simulink model "Citation"  (R2018a)
settings: Solver=ode5  StartTime=0.0  StopTime=500  FixedStep=0.01  RelTol=1e-3  EnableMultiTasking=on
InitFcn:
  | initcit
values from neighbouring files (symbols this model uses):
  aeroinit = [dp_ini;inicoef('CX0');inicoef('CXa');inicoef('CXa2');inicoef('CXq')     ;inicoef('CXde');inicoef('CY0');inicoef('CYB');inicoef('CYp');inicoef('CYr')     ;inicoef('CYda');inicoef('CYdr');inicoef('CZ0');inicoef('CZa');inicoef('CZq')     ;inicoef('CZde');inicoef('Cl0');inicoef('ClB');inicoef('Clp');inicoef('Clr')     ;inicoef('Clda');inicoef('Cldr');inicoef('Cm0');inicoef('Cma');inicoef('Cmq')     ; ...(+113 chars)    [initcit.m]
  h_l_old = zeros(6,sample_size)    [initcit.m]
  h_m_old = zeros(4,sample_size)    [initcit.m]
  h_n_old = zeros(6,sample_size)    [initcit.m]
  h_X_old = zeros(5,sample_size)    [initcit.m]
  h_Y_old = zeros(6,sample_size)    [initcit.m]
  h_Z_old = zeros(4,sample_size)    [initcit.m]
  I = [massinit(5),0, -massinit(8);0, massinit(6),0;-massinit(8),0, massinit(7)]    [initcit.m]
  p_l = [inicoef('Cl0');inicoef('ClB');inicoef('Clp');inicoef('Clr')     ;inicoef('Clda');inicoef('Cldr')].*ones(6,sample_size)    [initcit.m]
  p_m = [inicoef('Cm0');inicoef('Cma');inicoef('Cmq')     ;inicoef('Cmde')].*ones(4,sample_size)    [initcit.m]
  p_n = 0.71*ones(6,sample_size)    [initcit.m]
  p_X = [inicoef('CX0');inicoef('CXa');inicoef('CXa2');inicoef('CXq')     ;inicoef('CXde')].*ones(5,sample_size)    [initcit.m]
  p_Y = [inicoef('CY0');inicoef('CYB');inicoef('CYp');inicoef('CYr')     ;inicoef('CYda');inicoef('CYdr')].*ones(6,sample_size)    [initcit.m]
  p_Z = [inicoef('CZ0');inicoef('CZa');inicoef('CZq')     ;inicoef('CZde')].*ones(4,sample_size)    [initcit.m]
  Pcov_l = 10000*eye(6)    [initcit.m]
  Pcov_m = 10000*eye(4)    [initcit.m]
  Pcov_n = 10000*eye(6)    [initcit.m]
  Pcov_X = 10000*eye(5)    [initcit.m]
  Pcov_Y = 10000*eye(6)    [initcit.m]
  Pcov_Z = 10000*eye(4)    [initcit.m]
  T0 = 288.15    [rho_test.m]
  Vw915 = 0    [initcit.m]
  winddir = 45*(pi/180)    (= 0.785398163397)    [initcit.m]
  x0 = []    [cessnac550_3d_sfnc.m]    (also in sfunxyauto.m)
  y_l = zeros(1,sample_size)    [initcit.m]
  y_l_est_old = zeros(size(y_l))    [initcit.m]
  y_m = zeros(1,sample_size)    [initcit.m]
  y_m_est_old = zeros(size(y_m))    [initcit.m]
  y_n = zeros(1,sample_size)    [initcit.m]
  y_n_est_old = zeros(size(y_n))    [initcit.m]
  y_X = zeros(1,sample_size)    [initcit.m]
  y_X_est_old = zeros(size(y_X))    [initcit.m]
  y_Y = zeros(1,sample_size)    [initcit.m]
  y_Y_est_old = zeros(size(y_Y))    [initcit.m]
  y_Z = zeros(1,sample_size)    [initcit.m]
  y_Z_est_old = zeros(size(y_Z))    [initcit.m]
undefined symbols (not defined in the file or in its folder): chord, cv1, cv2, cv3, cv4, deltagmax1, deltagmax2, deltagmax3, deltagmax4, Deng, ealphag, ealphas, g0, hDME, hGS, kt1, kt2, kt3, lh, massinit, matbuaf, matdaf, matdam, matdbbf, matdeaf, matdgaf, matdqaf, matduaf, matdwaw, matedhr, mateif, matelhr, matemhr, matemv1, matemv2, matemve, matetam, mateuaf, matfaaf, matfaxl, matff, matibaf, matibb, matibmh, matipaf, matipmh, matiraf, matiuaf, matiwaf, matlaf, matlam, matleaf, matleam, matlgaf, matlqaf, matluaf, matmaaf, matmaam, matmaf, matmam ... (+75)
libraries: simulink x5, templibrary x3, vrlib x1
(part 2 of 6)

== system Citation/Aero Forces & Moments /Aerodynamic Moment Components/Cm ==
  "model output " : Inport
  Dynamic Pressure : Inport  Port=2
  Constant : Constant  Value=massinit
  Constant1 : Constant  Value=S
  Constant2 : Constant  Value=chord
  Demux2 : Demux  Outputs=[1 1 1 9 1 1 1 22]
  Demux3 : Demux  Outputs=[4 1 1 1 1]
  Divide : Product  Inputs=*/
  Product : Product  Inputs=3
  Product{1,3..5} (4 alike) : Product
  Product2 : Product  Inputs=3
  Sum : Sum  Inputs=|+++
  Sum1 : Sum  Inputs=|+-
  Sum2 : Sum  Inputs=|+-
  Terminator{1..6} (6 alike) : Terminator
  Cm : Outport
  wires:
  Demux3/4 -> Sum1/2  "Izz"
  Demux2/8 -> Terminator4/1
  Demux3/5 -> Product5/2  "Ixz"
  Demux2/7 -> Terminator6/1  "rdot"
  Demux2/1 -> Product3/2, Product3/1, Product2/1  "p"
  Demux2/6 -> Product1/1  "qdot"
  Demux3/2 -> Sum1/1  "Ixx"
  Demux2/4 -> Terminator3/1
  Demux3/1 -> Terminator5/1
  Demux2/5 -> Terminator2/1  "pdot"
  Demux3/3 -> Product1/2  "Iyy"
  "model output "/1 -> Demux2/1
  Constant/1 -> Demux3/1
  Sum/1 -> Divide/1
  Divide/1 -> Cm/1
  Dynamic Pressure/1 -> Product/1
  Constant1/1 -> Product/2
  Constant2/1 -> Product/3
  Product/1 -> Divide/2
  Product1/1 -> Sum/2  "qdot*Iyy"
  Sum1/1 -> Product2/3
  Demux2/2 -> Terminator1/1  "q"
  Demux2/3 -> Product4/2, Product4/1, Product2/2  "r"
  Product2/1 -> Sum/1  "rp*(Ixx-Izz)"
  Product3/1 -> Sum2/1  "p^2"
  Product4/1 -> Sum2/2  "r^2"
  Sum2/1 -> Product5/1
  Product5/1 -> Sum/3  "(p^2 - r^2)*(Ixz)"

== system Citation/Aero Forces & Moments /Aerodynamic Moment Components/Cn ==
  model output : Inport
  Dynamic Pressure : Inport  Port=2
  Constant : Constant  Value=massinit
  Constant1 : Constant  Value=S
  Constant2 : Constant  Value=span
  Demux2 : Demux  Outputs=[1 1 1 9 1 1 1 22]
  Demux3 : Demux  Outputs=[4 1 1 1 1]
  Divide : Product  Inputs=*/
  Product : Product  Inputs=3
  Product1 : Product
  Product2 : Product  Inputs=3
  Product3 : Product
  Product4 : Product
  Sum : Sum  Inputs=+++
  Sum1 : Sum  Inputs=|-+
  Sum2 : Sum  Inputs=|+-
  Terminator{1,3..5} (4 alike) : Terminator
  Cn : Outport
  wires:
  Demux3/4 -> Product1/2  "Izz"
  Demux2/8 -> Terminator4/1
  Demux3/5 -> Product3/2  "Ixz"
  Demux2/2 -> Product4/1, Product2/2  "q"
  Demux2/7 -> Product1/1  "rdot"
  Demux2/6 -> Terminator1/1  "qdot"
  Demux3/2 -> Sum1/1  "Ixx"
  Demux2/4 -> Terminator3/1
  Demux3/1 -> Terminator5/1
  Demux2/5 -> Sum2/2  "pdot"
  Demux3/3 -> Sum1/2  "Iyy"
  model output/1 -> Demux2/1
  Constant/1 -> Demux3/1
  Dynamic Pressure/1 -> Product/1
  Constant1/1 -> Product/2
  Constant2/1 -> Product/3
  Product/1 -> Divide/2  "0.5*rho*V^2*S*b"
  Sum/1 -> Divide/1  "rdot*Izz+pq*(Iyy-Ixx)+(qr-pdot)*Ixz"
  Product1/1 -> Sum/2  "rdot*Izz"
  Demux2/1 -> Product2/1  "p"
  Demux2/3 -> Product4/2  "r"
  Sum1/1 -> Product2/3
  Product2/1 -> Sum/1  "p*q*(Iyy-Ixx)"
  Product3/1 -> Sum/3  "Ixz*(qr-pdot)"
  Product4/1 -> Sum2/1
  Sum2/1 -> Product3/1
  Divide/1 -> Cn/1

== system Citation/Aerodynamic Parameter Estimation/Statistics 2/Auto_correlation ==
  delta_window : Inport
  kgap : Inport  Port=2
  Memory3 : Memory
  Memory4 : Memory
  autocorrelation : MATLAB Function  TreatAsAtomicUnit=on
  PI_kgap : Outport
  PI_kgap_avg : Outport  Port=2
  wires:
  kgap/1 -> autocorrelation/2(kgap)
  autocorrelation/3(counter) -> Memory4/1
  Memory4/1 -> autocorrelation/4("counter ")
  autocorrelation/1(PI_kgap) -> PI_kgap/1
  autocorrelation/2(kgap_avg) -> Memory3/1, PI_kgap_avg/1
  Memory3/1 -> autocorrelation/3("kgap_avg ")
  delta_window/1 -> autocorrelation/1(delta)

== system Citation/Aerodynamic Parameter Estimation/Statistics 2/variance ==
  delta : Inport
  MATLAB Function : MATLAB Function  TreatAsAtomicUnit=on
  Memory : Memory
  Memory1 : Memory
  Memory2 : Memory  InitialCondition=[0, 0]
  variance : Outport
  sigma_avg : Outport  Port=2
  wires:
  Memory1/1 -> MATLAB Function/2("delta_avg ")
  MATLAB Function/4(sigma_avg) -> sigma_avg/1, Memory2/1
  Memory2/1 -> MATLAB Function/4("sigma_avg ")
  MATLAB Function/2(delta_avg) -> Memory1/1  "average"
  Memory/1 -> MATLAB Function/3("counter ")
  MATLAB Function/1(var) -> variance/1
  MATLAB Function/3(counter) -> Memory/1
  delta/1 -> MATLAB Function/1(delta)

== system Citation/Aerodynamic Parameter Estimation/Statistics 3/Auto_correlation ==
  delta_window : Inport
  kgap : Inport  Port=2
  Memory3 : Memory
  Memory4 : Memory
  autocorrelation : MATLAB Function  TreatAsAtomicUnit=on
  PI_kgap : Outport
  PI_kgap_avg : Outport  Port=2
  wires:
  delta_window/1 -> autocorrelation/1(delta)
  Memory3/1 -> autocorrelation/3("kgap_avg ")
  autocorrelation/2(kgap_avg) -> PI_kgap_avg/1, Memory3/1
  autocorrelation/1(PI_kgap) -> PI_kgap/1
  Memory4/1 -> autocorrelation/4("counter ")
  autocorrelation/3(counter) -> Memory4/1
  kgap/1 -> autocorrelation/2(kgap)

== system Citation/Aerodynamic Parameter Estimation/Statistics 3/variance ==
  delta : Inport
  MATLAB Function : MATLAB Function  TreatAsAtomicUnit=on
  Memory : Memory
  Memory1 : Memory
  Memory2 : Memory  InitialCondition=[0, 0]
  variance : Outport
  sigma_avg : Outport  Port=2
  wires:
  delta/1 -> MATLAB Function/1(delta)
  MATLAB Function/3(counter) -> Memory/1
  MATLAB Function/1(var) -> variance/1
  Memory/1 -> MATLAB Function/3("counter ")
  MATLAB Function/2(delta_avg) -> Memory1/1  "average"
  Memory2/1 -> MATLAB Function/4("sigma_avg ")
  MATLAB Function/4(sigma_avg) -> Memory2/1, sigma_avg/1
  Memory1/1 -> MATLAB Function/2("delta_avg ")

== system Citation/Aerodynamic Parameter Estimation/Statistics 4/Auto_correlation ==
  delta_window : Inport
  kgap : Inport  Port=2
  Memory3 : Memory
  Memory4 : Memory
  autocorrelation : MATLAB Function  TreatAsAtomicUnit=on
  PI_kgap : Outport
  PI_kgap_avg : Outport  Port=2
  wires:
  kgap/1 -> autocorrelation/2(kgap)
  autocorrelation/3(counter) -> Memory4/1
  Memory4/1 -> autocorrelation/4("counter ")
  autocorrelation/1(PI_kgap) -> PI_kgap/1
  autocorrelation/2(kgap_avg) -> Memory3/1, PI_kgap_avg/1
  Memory3/1 -> autocorrelation/3("kgap_avg ")
  delta_window/1 -> autocorrelation/1(delta)

== system Citation/Aerodynamic Parameter Estimation/Statistics 4/variance ==
  delta : Inport
  MATLAB Function : MATLAB Function  TreatAsAtomicUnit=on
  Memory : Memory
  Memory1 : Memory
  Memory2 : Memory  InitialCondition=[0, 0]
  variance : Outport
  sigma_avg : Outport  Port=2
  wires:
  Memory1/1 -> MATLAB Function/2("delta_avg ")
  MATLAB Function/4(sigma_avg) -> sigma_avg/1, Memory2/1
  Memory2/1 -> MATLAB Function/4("sigma_avg ")
  MATLAB Function/2(delta_avg) -> Memory1/1  "average"
  Memory/1 -> MATLAB Function/3("counter ")
  MATLAB Function/1(var) -> variance/1
  MATLAB Function/3(counter) -> Memory/1
  delta/1 -> MATLAB Function/1(delta)

== system Citation/Cessna Citation 500/Actuators/da ==
  In : Inport
  Gain : Gain  Gain=13  SaturateOnIntegerOverflow=on  OutDataTypeStr=Inherit: Same as input  ParamDataTypeStr=Inherit: Same as input
  Integrator : Integrator  InitialCondition=u0(2)
  Sum : Sum  Inputs=|+-  SaturateOnIntegerOverflow=on
  Out : Outport
  wires:
  Integrator/1 -> Out/1, Sum/2
  In/1 -> Sum/1
  Sum/1 -> Gain/1
  Gain/1 -> Integrator/1

== system Citation/Cessna Citation 500/Actuators/de ==
  In : Inport
  Gain : Gain  Gain=13  SaturateOnIntegerOverflow=on  OutDataTypeStr=Inherit: Same as input  ParamDataTypeStr=Inherit: Same as input
  Integrator : Integrator  InitialCondition=u0(1)
  Sum : Sum  Inputs=|+-  SaturateOnIntegerOverflow=on
  Out : Outport
  wires:
  Integrator/1 -> Out/1, Sum/2
  In/1 -> Sum/1
  Sum/1 -> Gain/1
  Gain/1 -> Integrator/1

== system Citation/Cessna Citation 500/Actuators/dr ==
  In : Inport
  Gain : Gain  Gain=13  SaturateOnIntegerOverflow=on  OutDataTypeStr=Inherit: Same as input  ParamDataTypeStr=Inherit: Same as input
  Integrator : Integrator  InitialCondition=u0(3)
  Sum : Sum  Inputs=|+-  SaturateOnIntegerOverflow=on
  Out : Outport
  wires:
  Integrator/1 -> Out/1, Sum/2
  In/1 -> Sum/1
  Sum/1 -> Gain/1
  Gain/1 -> Integrator/1

== system Citation/Cessna Citation 500/Actuators/flaps ==
  In : Inport
  Gain : Gain  Gain=0.9  SaturateOnIntegerOverflow=on  OutDataTypeStr=Inherit: Same as input  ParamDataTypeStr=Inherit: Same as input
  Integrator : Integrator  InitialCondition=u0(7)
  Sum : Sum  Inputs=|+-  SaturateOnIntegerOverflow=on
  Out : Outport
  wires:
  Integrator/1 -> Out/1, Sum/2
  In/1 -> Sum/1
  Sum/1 -> Gain/1
  Gain/1 -> Integrator/1

== system Citation/Cessna Citation 500/Actuators/gear ==
  In : Inport
  Gain : Gain  Gain=0.6  SaturateOnIntegerOverflow=on  OutDataTypeStr=Inherit: Same as input  ParamDataTypeStr=Inherit: Same as input
  Integrator : Integrator  InitialCondition=u0(8)
  Sum : Sum  Inputs=|+-  SaturateOnIntegerOverflow=on
  Out : Outport
  wires:
  Integrator/1 -> Out/1, Sum/2
  In/1 -> Sum/1
  Sum/1 -> Gain/1
  Gain/1 -> Integrator/1

== system Citation/Cessna Citation 500/Citation model DASMAT/AIRCRAFT MODEL ==
  ua : Inport
  ut : Inport  Port=2
  massinit : Inport  Port=3
  Environment : Inport  Port=4
  AFM : Subsystem
  AIRDATA : Subsystem
  Demux : Demux  Outputs=[8 1]
  EFM : Subsystem
  EQM : Subsystem
  FM SORT : Subsystem
  GRAVITY : Subsystem
  LANDING GEAR : Subsystem
  OBSERVATIONS : Subsystem
  WIND/TURBULENCE : Subsystem
  x : Outport
  xdot : Outport  Port=2
  yatm : Outport  Port=3
  yad1 : Outport  Port=4
  yad2 : Outport  Port=5
  wind : Outport  Port=6
  gust : Outport  Port=7
  yacc : Outport  Port=8
  yfp : Outport  Port=9
  ys : Outport  Port=10
  FMa : Outport  Port=11
  FMag : Outport  Port=12
  FMt : Outport  Port=13
  ypp : Outport  Port=14
  wires:
  AFM/1(FMa) -> FM SORT/1(FMa), EQM/2(FMa)
  OBSERVATIONS/3(ys) -> ys/1
  OBSERVATIONS/2(yfp) -> yfp/1
  EQM/4(FMtot corrected) -> OBSERVATIONS/4(FMtot)
  EQM/3(yuvw) -> OBSERVATIONS/3(yuvw)
  EFM/1(FMt) -> FM SORT/3(FMt), FMt/1
  AFM/4(FMag) -> FM SORT/2(FMag), FMag/1
  ua/1 -> AFM/2(ua), LANDING GEAR/4(ua)
  ut/1 -> EFM/2(ut)
  OBSERVATIONS/1(yacc) -> yacc/1
  FM SORT/1(FMtot) -> EQM/1("FMtot ")
  EQM/5(FMa corrected) -> OBSERVATIONS/5(FMa), FMa/1
  AFM/2(FMadot) -> EQM/3(FMadot)
  AFM/3(FMbdot) -> EQM/4(FMbdot)
  GRAVITY/1(Fgr) -> FM SORT/4("Fgr "), OBSERVATIONS/6(Fgr)
  massinit/1 -> EFM/3(massinit), AFM/3(massinit), GRAVITY/2(massinit), EQM/5(massinit), OBSERVATIONS/7(massinit), LANDING GEAR/3(massinit)
  AIRDATA/3(yad2) -> EFM/6(yad2), AFM/5(yad2), yad2/1
  AIRDATA/2(yad1) -> AFM/4(yad1), EFM/5(yad1), yad1/1
  AIRDATA/1(yatm) -> yatm/1, GRAVITY/3(yatm), OBSERVATIONS/8(yatm), EFM/4(yatm), AFM/7(yatm)
  EQM/1(x) -> GRAVITY/1("x "), LANDING GEAR/1(x), EFM/1(x), AFM/1(x), WIND/TURBULENCE/1("x "), AIRDATA/1(x), x/1, OBSERVATIONS/1(x)
  WIND/TURBULENCE/1(wind) -> EQM/6(wind), wind/1
  EQM/2(xdot) -> xdot/1, OBSERVATIONS/2(xdot), LANDING GEAR/2(xdot)
  Environment/1 -> Demux/1
  Demux/1 -> gust/1, AFM/6(gust)
  Demux/2 -> AIRDATA/2(terrain elevation), LANDING GEAR/5(terr elev)  "terrain elevation"
  LANDING GEAR/1(Fmt) -> FM SORT/5(Fgear)
  EFM/2(ypp) -> ypp/1

== system Citation/Cessna Citation 500/Controllers/NDI rotational rate controller ==
  note: 1st order filters
  note: And scale to max angular rates
  note: normalize inputs back from deflection values
  note: u=b^-1(v-a)
  note: correct order
  note: p
      | q
      | r
      | vtas
      | alpha
      | beta
      | phi
      | theta
      | psi
      | he
      | xe
      | ye
  note: de
      | da
      | dr
      | dte
      | dta
      | dtr
      | df
      | gear
      | pla1
      | pla2
  note: [1]
  note: Cl0
      | ClB
      | Clp
      | Clr
      | Clda
      | Cldr
  note: dynamic pressure
  note: CZ0
      | CZa
      | CZq
      | CZde
  note: CY0
      | CYB
      | CYp
      | CYr
      | CYda
      | CYdr
  note: Cn0
      | CnB
      | Cnp
      | Cnr
      | Cnda
      | Cndr
  note: CX0
      | CXa
      | CXa^2
      | CXq
      | CXde
  note: Cm0
      | Cma
      | Cmq
      | Cmde
  note: [23:26]
  note: [13:16]
  note: [27:32]
  note: [17:22]
  note: [7:12]
  note: [2:6]
  note: Aerodata Description
  note: correct order
  note: de
      | da
      | dr
      | dte
      | dta
      | dtr
      | df
      | gear
      | pla1
      | pla2
  inputs : Inport
  A/C state : Inport  Port=2
  aero data : Inport  Port=3
  Demux : Demux  Outputs=[1 1 1 7]
  Demux1 : Demux  Outputs=[3 2 1 6]
  Demux2 : Demux  Outputs=3
  Demux3 : Demux  Outputs=3
  Demux4 : Demux  Commented=on  Outputs=3
  Gain1 : Gain  Gain=-1  SaturateOnIntegerOverflow=on  OutDataTypeStr=Inherit: Same as input  ParamDataTypeStr=Inherit: Same as input
  Gain10 : Gain  Gain=180/pi  SaturateOnIntegerOverflow=on  OutDataTypeStr=Inherit: Same as input  ParamDataTypeStr=Inherit: Same as input
  Gain11 : Gain  Gain=180/pi  SaturateOnIntegerOverflow=on  OutDataTypeStr=Inherit: Same as input  ParamDataTypeStr=Inherit: Same as input
  Gain12 : Gain  Gain=0.5  SaturateOnIntegerOverflow=on  OutDataTypeStr=Inherit: Same as input  ParamDataTypeStr=Inherit: Same as input
  Gain2 : Gain  Gain=-1  SaturateOnIntegerOverflow=on  OutDataTypeStr=Inherit: Same as input  ParamDataTypeStr=Inherit: Same as input
  Gain3 : Gain  Gain=4  SaturateOnIntegerOverflow=on  OutDataTypeStr=Inherit: Same as input  ParamDataTypeStr=Inherit: Same as input
  Gain4 : Gain  Gain=-1  SaturateOnIntegerOverflow=on  OutDataTypeStr=Inherit: Same as input  ParamDataTypeStr=Inherit: Same as input
  Gain5 : Gain  Gain=1/37.24  SaturateOnIntegerOverflow=on  OutDataTypeStr=Inherit: Same as input  ParamDataTypeStr=Inherit: Same as input
  Gain6 : Gain  Gain=1/20  SaturateOnIntegerOverflow=on  OutDataTypeStr=Inherit: Same as input  ParamDataTypeStr=Inherit: Same as input
  Gain7 : Gain  Gain=1.5  SaturateOnIntegerOverflow=on  OutDataTypeStr=Inherit: Same as input  ParamDataTypeStr=Inherit: Same as input
  Gain8 : Gain  Gain=1/22  SaturateOnIntegerOverflow=on  OutDataTypeStr=Inherit: Same as input  ParamDataTypeStr=Inherit: Same as input
  Gain9 : Gain  Gain=180/pi  SaturateOnIntegerOverflow=on  OutDataTypeStr=Inherit: Same as input  ParamDataTypeStr=Inherit: Same as input
  Linear Controller : Subsystem
  Memory : Memory  InitialCondition=eye(3)
  Mux : Mux  Inputs=3
  Mux1 : Mux
  Sum : Sum  Inputs=|+-
  Sum1 : Sum  Inputs=|+-
  Terminator1 : Terminator
  Terminator2 : Terminator
  Time Scope : Scope  NumInputPorts=3
  Time Scope1 : Scope  NumInputPorts=3
  Time Scope2 : Scope  Commented=on  NumInputPorts=3
  Time Scope3 : Scope  NumInputPorts=3
  Transfer Fcn : TransferFcn  Denominator=[0.1 1]
  Transfer Fcn1 : TransferFcn  Denominator=[0.1 1]
  Transfer Fcn2 : TransferFcn  Denominator=[0.1 1]
  a : MATLAB Function  TreatAsAtomicUnit=on
  b^-1 : MATLAB Function  TreatAsAtomicUnit=on
  da limits : Saturate  UpperLimit=0.65  LowerLimit=-0.65
  de limits : Saturate  UpperLimit=0.26  LowerLimit=-0.35
  dr limits : Saturate  UpperLimit=0.38  LowerLimit=-0.38
  control input : Outport
  wires:
  Transfer Fcn2/1 -> Time Scope/3, Mux/3  "rref"
  Transfer Fcn1/1 -> Time Scope/1, Mux/1  "pref"
  Transfer Fcn/1 -> Time Scope/2, Mux/2  "qref"
  inputs/1 -> Demux/1
  Sum/1 -> Demux3/1, Linear Controller/1(e_omega)
  Demux1/2 -> Terminator1/1
  Demux1/1 -> Demux4/1, Sum/2  "p q r"
  A/C state/1 -> a/2(state), Demux1/1
  Mux1/1 -> control input/1
  aero data/1 -> b^-1/2(aerodat), a/1(aerodat)
  b^-1/2(mat_old) -> Memory/1
  Memory/1 -> b^-1/3("mat_old ")
  Demux/4 -> [RC]
  [RC] -> Mux1/4
  Demux2/2 -> de limits/1  "de"
  Demux2/1 -> da limits/1  "da"
  Demux2/3 -> dr limits/1  "dr"
  a/1(y) -> Sum1/2
  Linear Controller/1(v) -> Sum1/1  "vp vq vr"
  Sum1/1 -> b^-1/1(ve)
  b^-1/1(delta) -> Demux2/1  "da de dr"
  Mux/1 -> Sum/1  "pref qref rref"
  Demux/1 -> Gain2/1
  Demux/2 -> Gain1/1
  Gain8/1 -> Gain11/1
  Gain4/1 -> Gain8/1
  Gain1/1 -> Gain5/1
  Gain2/1 -> Gain6/1
  Gain5/1 -> Gain9/1
  Gain6/1 -> Gain10/1
  Demux/3 -> Gain4/1
  Demux3/1 -> Time Scope1/1
  Demux3/2 -> Time Scope1/2
  Demux3/3 -> Time Scope1/3
  Demux4/3 -> Time Scope2/3
  Demux4/2 -> Time Scope2/2
  Demux4/1 -> Time Scope2/1
  Gain9/1 -> Gain3/1
  Gain3/1 -> Transfer Fcn1/1
  Gain11/1 -> Gain12/1
  Gain12/1 -> Transfer Fcn2/1
  Gain10/1 -> Gain7/1
  Gain7/1 -> Transfer Fcn/1
  de limits/1 -> Time Scope3/2, Mux1/1
  da limits/1 -> Time Scope3/1, Mux1/2
  dr limits/1 -> Time Scope3/3, Mux1/3
  Demux1/4 -> Terminator2/1

== system Citation/Cessna Citation 500/Controllers/Yaw damper ==
  state : Inport
  inputs : Inport  Port=2
  Gain : Gain  SaturateOnIntegerOverflow=on  OutDataTypeStr=Inherit: Same as input  ParamDataTypeStr=Inherit: Same as input
  Washout : TransferFcn  Numerator=[1 0]  Denominator=[1 1/4]
  dr : Gain  Gain=[0 0 1 0 0 0 0 0 0 0]  SaturateOnIntegerOverflow=on  OutDataTypeStr=Inherit: Same as input  ParamDataTypeStr=Inherit: Same as input
  not used : Terminator
  r  sel : Selector  IndexOptions=Index vector (dialog)  Indices=[3]  OutputSizes=1
  controller output : Outport
  wires:
  Washout/1 -> Gain/1
  dr/1 -> controller output/1
  state/1 -> r  sel/1
  r  sel/1 -> Washout/1  "r"
  inputs/1 -> not used/1
  Gain/1 -> dr/1

== system Citation/Cessna Citation 500/Controllers/auto throttle ==
  state : Inport
  inputs : Inport  Port=2
  Gain : Gain  Gain=0.5  SaturateOnIntegerOverflow=on  OutDataTypeStr=Inherit: Same as input  ParamDataTypeStr=Inherit: Same as input
  Saturation : Saturate  UpperLimit=1.0  LowerLimit=0.0
  Sum : Sum  Inputs=+-|  SaturateOnIntegerOverflow=on
  VTAS ref (trim value) : Constant  Value=x0(4)
  VTAS sel : Selector  IndexOptions=Index vector (dialog)  Indices=[4]  OutputSizes=1
  controller output is later added to pilot input! : Sum  Inputs=|+-  SaturateOnIntegerOverflow=on
  pla1&2 : Gain  Gain=[0 0 0 0 0 0 0 0 1 1]  SaturateOnIntegerOverflow=on  OutDataTypeStr=Inherit: Same as input  ParamDataTypeStr=Inherit: Same as input
  pla1&2 as well : Gain  Gain=[0 0 0 0 0 0 0 0 1 1]  SaturateOnIntegerOverflow=on  OutDataTypeStr=Inherit: Same as input  ParamDataTypeStr=Inherit: Same as input
  controller output : Outport
  wires:
  inputs/1 -> pla1&2 as well/1
  state/1 -> VTAS sel/1
  VTAS sel/1 -> Sum/2  "VTAS"
  VTAS ref (trim value)/1 -> Sum/1
  Sum/1 -> Gain/1
  pla1&2/1 -> controller output is later added to pilot input!/1
  Gain/1 -> Saturation/1
  controller output is later added to pilot input!/1 -> controller output/1
  Saturation/1 -> pla1&2/1
  pla1&2 as well/1 -> controller output is later added to pilot input!/2

== system Citation/Cessna Citation 500/Controllers/beta feedback ==
  note: elevator [-0.6973,-0.033,0.5725] backwards+
  note: p
      | q
      | r
      | vtas
      | alpha
      | beta
      | phi
      | theta
      | psi
      | he
      | xe
      | ye
  state : Inport
  input : Inport  Port=2
  Demux : Demux  Commented=on  Outputs=[1 1 2 1 2 1 4]
  Demux1 : Demux  Outputs=[5 1 6]
  Gain : Gain  Commented=on  Gain=[1 0 0 0 0 0 0 0 0 0]
  Gain1 : Gain  Commented=on  Gain=-1
  PID Controller1 : simulink/Continuous/PID Controller  Commented=on  Controller=PID  TimeDomain=Continuous-time  SampleTime=-1  IntegratorMethod=Forward Euler  FilterMethod=Forward Euler  Form=Parallel  UseFilter=on  ControllerParametersSource=internal  P=1  I=50  D=5  N=1  InitialConditionSource=internal  InitialConditionForIntegrator=0  InitialConditionForFilter=0  ExternalReset=none  LimitOutput=off  UpperSaturationLimit=inf  LowerSaturationLimit=-inf  LinearizeAsGain=on  AntiWindupMode=none  Kb=1  TrackingMode=off  Kt=1  PParamMin=[]  PParamMax=[]  IParamMin=[]  IParamMax=[]  DParamMin=[]  DParamMax=[]  NParamMin=[]  NParamMax=[]  KbParamMin=[]  KbParamMax=[]  KtParamMin=[]  KtParamMax=[]  POutMin=[]  POutMax=[]  IOutMin=[]  IOutMax=[]  DOutMin=[]  DOutMax=[]  NOutMin=[]  NOutMax=[]  KbOutMin=[]  KbOutMax=[]  KtOutMin=[]  KtOutMax=[]  IntegratorOutMin=[]  IntegratorOutMax=[]  FilterOutMin=[]  FilterOutMax=[]  SumOutMin=[]  SumOutMax=[]  SumI1OutMin=[]  SumI1OutMax=[]  SumI2OutMin=[]  SumI2OutMax=[]  SumI3OutMin=[]  SumI3OutMax=[]  SumDOutMin=[]  SumDOutMax=[]  SaturationOutMin=[]  SaturationOutMax=[]  IntegratorContinuousStateAttributes=''  IntegratorStateMustResolveToSignalObject=off  IntegratorRTWStateStorageClass=Auto  FilterContinuousStateAttributes=''  FilterStateMustResolveToSignalObject=off  FilterRTWStateStorageClass=Auto  DifferentiatorICPrevScaledInput=0  DifferentiatorOutMin=[]  DifferentiatorOutMax=[]  FilterDiffOutCoefMin=[]  FilterDiffOutCoefMax=[]  SumDenOutMin=[]  SumDenOutMax=[]  SumNumOutMin=[]  SumNumOutMax=[]  ReciprocalOutMin=[]  ReciprocalOutMax=[]  DivideOutMin=[]  DivideOutMax=[]  TunerSelectOption=Transfer Function Based (PID Tuner App)
  Sum : Sum  Commented=on  Inputs=|+-
  Sum1 : Sum  Commented=on  Inputs=|-+
  Terminator{,1..3} (4 alike) : Terminator  Commented=on
  Time Scope : Scope  Commented=on
  Transfer Fcn : TransferFcn  Commented=on  Numerator=[1 0]  Denominator=[1 1/4]
  gamma_r : Constant  Commented=on  Value=-0.033
  Out1 : Outport
  wires:
  gamma_r/1 -> Sum/1
  state/1 -> Demux1/1, Demux/1
  Demux/1 -> Terminator/1
  Demux/3 -> Terminator1/1
  Demux/5 -> Terminator2/1
  Demux/7 -> Terminator3/1
  Demux/2 -> ?  "q"
  Demux/4 -> Sum1/1  "alpha"
  Demux/6 -> Sum1/2  "theta"
  Sum1/1 -> Sum/2  "gamma"
  Sum/1 -> Gain1/1
  Transfer Fcn/1 -> Time Scope/1, Gain/1
  Gain1/1 -> PID Controller1/1
  PID Controller1/1 -> Transfer Fcn/1
  Demux1/2 -> ?

== system Citation/Pilot/Joystick/DualShock ==
  note: Apply Dead zone
  note: Currently configured for a Sony Dualshock 3 Playstation 3 Controller
  JoyStick input : Inport
  "Add deadzone " : Subsystem
  Add deadzone 1 : Subsystem
  Add deadzone 2 : Subsystem
  Add deadzone 3 : Subsystem
  Constant{,1..3} (4 alike) : Constant  Value=0
  Constant{4..7} (4 alike) : Constant  Value=0.05
  Dead Zone{,1..3} (4 alike) : DeadZone  LowerValue=-0.05  UpperValue=0.05  SaturateOnIntegerOverflow=on
  Demux : Demux  Outputs=[5 10]
  Demux1 : Demux  Outputs=5
  Demux2 : Demux  Outputs=[2 1 7]
  Display{,1..3} (4 alike) : Display
  Gain{,1..3} (4 alike) : Gain  Gain=-1  SaturateOnIntegerOverflow=on  OutDataTypeStr=Inherit: Same as input  ParamDataTypeStr=Inherit: Same as input
  Gain11 : Gain  Gain=pi/180  SaturateOnIntegerOverflow=on  OutDataTypeStr=Inherit: Same as input  ParamDataTypeStr=Inherit: Same as input
  Gain4 : Gain  Gain=37.24  SaturateOnIntegerOverflow=on  OutDataTypeStr=Inherit: Same as input  ParamDataTypeStr=Inherit: Same as input
  Gain5 : Gain  Gain=20  SaturateOnIntegerOverflow=on  OutDataTypeStr=Inherit: Same as input  ParamDataTypeStr=Inherit: Same as input
  Gain6 : Gain  SaturateOnIntegerOverflow=on  OutDataTypeStr=Inherit: Same as input  ParamDataTypeStr=Inherit: Same as input
  Gain7 : Gain  Gain=22  SaturateOnIntegerOverflow=on  OutDataTypeStr=Inherit: Same as input  ParamDataTypeStr=Inherit: Same as input
  Gain8 : Gain  Gain=pi/180  SaturateOnIntegerOverflow=on  OutDataTypeStr=Inherit: Same as input  ParamDataTypeStr=Inherit: Same as input
  Gain9 : Gain  Gain=pi/180  SaturateOnIntegerOverflow=on  OutDataTypeStr=Inherit: Same as input  ParamDataTypeStr=Inherit: Same as input
  Mux : Mux  Inputs=5
  Sum{,1..3} (4 alike) : Sum  Inputs=-+|  SaturateOnIntegerOverflow=on
  Terminator : Terminator
  Terminator1 : Terminator
  Terminator2 : Terminator
  "Model Input " : Outport
  wires:
  Gain3/1 -> Gain7/1
  Constant4/1 -> "Add deadzone "/1("Value ")
  Gain4/1 -> Gain8/1
  Constant5/1 -> Add deadzone 3/1("Value ")
  Constant/1 -> Sum/1
  Sum3/1 -> Dead Zone2/1
  "Add deadzone "/1(Out1) -> Gain/1
  Demux1/3 -> Terminator/1
  Demux1/4 -> Sum3/2
  Dead Zone/1 -> "Add deadzone "/2("Input ")
  Sum2/1 -> Dead Zone3/1
  Gain8/1 -> Mux/1, Display/1
  Dead Zone1/1 -> Add deadzone 1/2("Input ")
  Demux1/5 -> Sum1/2
  Add deadzone 1/1(Out1) -> Gain1/1
  Add deadzone 3/1(Out1) -> Gain3/1
  Constant1/1 -> Sum1/1
  Demux1/2 -> Sum2/2
  Gain5/1 -> Gain9/1
  Gain11/1 -> Mux/4, Display3/1
  Constant3/1 -> Sum3/1
  Gain1/1 -> Gain5/1
  Dead Zone2/1 -> Add deadzone 3/2("Input ")
  Add deadzone 2/1(Out1) -> Gain2/1
  Gain/1 -> Gain4/1
  Dead Zone3/1 -> Add deadzone 2/2("Input ")
  Sum/1 -> Dead Zone/1
  Gain9/1 -> Mux/2, Display2/1
  Constant7/1 -> Add deadzone 1/1("Value ")
  Constant6/1 -> Add deadzone 2/1("Value ")
  Sum1/1 -> Dead Zone1/1
  Gain6/1 -> Mux/3, Display1/1
  Gain7/1 -> Gain11/1
  Demux1/1 -> Sum/2
  Constant2/1 -> Sum2/1
  Gain2/1 -> Gain6/1
  JoyStick input/1 -> Demux/1
  Demux2/3 -> Terminator2/1
  Demux/2 -> Demux2/1  "buttons"
  Demux2/1 -> Terminator1/1
  Demux/1 -> Demux1/1
  Mux/1 -> "Model Input "/1
  Demux2/2 -> Mux/5

== system Citation/Pilot/Joystick/Logitech 3D Pro ==
  note: Apply Dead zone
  note: apply real limits
      | [deg]
      | [%]
  note: normalize inputs
      | aileron [-1,0,1] left+
      | elevator [-1,0,1] forward+
      | rudder [-1,0,1] left+
      | throttle [-1,0,1] forward+
  note: Convert to radians
      | [rad]
      | [%]
  note: raw inputs
      | aileron [-0.6328,0.014,0.72] right+
      | elevator [-0.6973,-0.033,0.5725] backwards+
      | throttle [-0.6407,0,0.5317]bacwards+
      | rudder [-0.56,0.127,0.73] right+
  note: Add Deadzone values
  note: Currently configured for a Logitech Xtreme 3D Pro Joystick
  "JoyStick Input " : Inport
  "Add deadzone " : Subsystem
  Add deadzone 1 : Subsystem
  Add deadzone 2 : Subsystem
  Add deadzone 3 : Subsystem
  Constant{,1..3,6} (5 alike) : Constant  Value=0
  Constant4 : Constant  Value=0.008
  Constant5 : Constant  Value=0.05
  Constant7 : Constant  Value=0.008
  Dead Zone : DeadZone  LowerValue=-0.008  UpperValue=0.008  SaturateOnIntegerOverflow=on
  Dead Zone1 : DeadZone  LowerValue=-0.008  UpperValue=0.008  SaturateOnIntegerOverflow=on
  Dead Zone2 : DeadZone  LowerValue=-0.05  UpperValue=0.05  SaturateOnIntegerOverflow=on
  Dead Zone3 : DeadZone  LowerValue=0  UpperValue=0  SaturateOnIntegerOverflow=on
  Demux : Demux  Outputs=[4 1 5 1 1]
  Demux1 : Demux
  Demux2 : Demux  Outputs=[4 12]
  Gain{,1..3} (4 alike) : Gain  Gain=-1  SaturateOnIntegerOverflow=on  OutDataTypeStr=Inherit: Same as input  ParamDataTypeStr=Inherit: Same as input
  Gain11 : Gain  Gain=pi/180  SaturateOnIntegerOverflow=on  OutDataTypeStr=Inherit: Same as input  ParamDataTypeStr=Inherit: Same as input
  Gain4 : Gain  Gain=37.24  SaturateOnIntegerOverflow=on  OutDataTypeStr=Inherit: Same as input  ParamDataTypeStr=Inherit: Same as input
  Gain5 : Gain  Gain=20  SaturateOnIntegerOverflow=on  OutDataTypeStr=Inherit: Same as input  ParamDataTypeStr=Inherit: Same as input
  Gain6 : Gain  SaturateOnIntegerOverflow=on  OutDataTypeStr=Inherit: Same as input  ParamDataTypeStr=Inherit: Same as input
  Gain7 : Gain  Gain=22  SaturateOnIntegerOverflow=on  OutDataTypeStr=Inherit: Same as input  ParamDataTypeStr=Inherit: Same as input
  Gain8 : Gain  Gain=pi/180  SaturateOnIntegerOverflow=on  OutDataTypeStr=Inherit: Same as input  ParamDataTypeStr=Inherit: Same as input
  Gain9 : Gain  Gain=pi/180  SaturateOnIntegerOverflow=on  OutDataTypeStr=Inherit: Same as input  ParamDataTypeStr=Inherit: Same as input
  Mux : Mux  Inputs=6
  Sum{,1..3} (4 alike) : Sum  Inputs=-+|  SaturateOnIntegerOverflow=on
  Terminator1 : Terminator
  Terminator2 : Terminator
  Terminator3 : Terminator
  Model Input : Outport
  wires:
  Constant1/1 -> Sum1/1
  Dead Zone3/1 -> Add deadzone 2/2("Input ")
  Sum2/1 -> Dead Zone3/1
  Constant6/1 -> Add deadzone 2/1("Value ")
  Sum/1 -> Dead Zone/1
  "Add deadzone "/1(Out1) -> Gain/1
  Constant7/1 -> Add deadzone 1/1("Value ")
  Add deadzone 3/1(Out1) -> Gain3/1
  Add deadzone 2/1(Out1) -> Gain2/1
  Gain5/1 -> Gain9/1
  Gain7/1 -> Gain11/1
  Constant4/1 -> "Add deadzone "/1("Value ")
  Add deadzone 1/1(Out1) -> Gain1/1
  Dead Zone2/1 -> Add deadzone 3/2("Input ")
  Constant2/1 -> Sum2/1
  Constant5/1 -> Add deadzone 3/1("Value ")
  Sum1/1 -> Dead Zone1/1
  Sum3/1 -> Dead Zone2/1
  Gain4/1 -> Gain8/1
  Demux1/1 -> Sum/2
  Dead Zone/1 -> "Add deadzone "/2("Input ")
  Gain1/1 -> Gain5/1
  Constant/1 -> Sum/1
  Demux2/1 -> Demux1/1  "axes"
  Dead Zone1/1 -> Add deadzone 1/2("Input ")
  Gain3/1 -> Gain7/1
  Constant3/1 -> Sum3/1
  Gain2/1 -> Gain6/1
  Gain/1 -> Gain4/1
  Demux1/3 -> Sum3/2
  Demux1/2 -> Sum1/2
  Demux1/4 -> Sum2/2
  Gain9/1 -> Mux/2  "elevator"
  Gain6/1 -> Mux/3  "thrust"
  Demux/3 -> Terminator2/1
  Demux/1 -> Terminator1/1
  Demux/2 -> Mux/5  "failure button"
  Demux2/2 -> Demux/1  "buttons"
  "JoyStick Input "/1 -> Demux2/1
  Mux/1 -> Model Input/1
  Gain8/1 -> Mux/1  "aileron"
  Gain11/1 -> Mux/4  "rudder"
  Demux/5 -> Terminator3/1
  Demux/4 -> Mux/6  "NDI toggle"

== system Citation/Pilot/button2toggle /Triggered Subsystem ==
  In1 : Inport
  Trigger : TriggerPort  VariantControl=Variant
  Out1 : Outport
  wires:
  In1/1 -> Out1/1

== system Citation/Pilot/button2toggle 1/Triggered Subsystem ==
  In1 : Inport
  Trigger : TriggerPort  VariantControl=Variant
  Out1 : Outport
  wires:
  In1/1 -> Out1/1

== system Citation/Cessna Citation 500/Citation model DASMAT/AIRCRAFT MODEL/AFM ==
  x : Inport
  ua : Inport  Port=2
  massinit : Inport  Port=3
  yad1 : Inport  Port=4
  yad2 : Inport  Port=5
  gust : Inport  Port=6
  yatm : Inport  Port=7
  Aero axes-cg transformation : Subsystem
  Aeromod : Subsystem
  FMaerodims : Subsystem
  FMgustdims : Subsystem
  Gust axes-cg transformation : Subsystem
  FMa : Outport
  FMadot : Outport  Port=2
  FMbdot : Outport  Port=3
  FMag : Outport  Port=4
  wires:
  FMaerodims/3(FMbdot) -> FMbdot/1
  FMgustdims/1(FMag) -> FMag/1
  FMaerodims/2(FMadot) -> FMadot/1
  FMaerodims/1(FMa) -> FMa/1
  ua/1 -> Aeromod/2(ua)
  yad2/1 -> Aeromod/5(yad2)
  gust/1 -> Aeromod/6(gust)
  Aero axes-cg transformation/1(Ca) -> FMaerodims/1(Ca)
  Aero axes-cg transformation/2(Cadot) -> FMaerodims/2(Cadot)
  Aero axes-cg transformation/3(Cbdot) -> FMaerodims/3(Cbdot)
  Gust axes-cg transformation/1(Cag) -> FMgustdims/1(Cag)
  yad1/1 -> FMaerodims/5(yad1), FMgustdims/2(yad1), Aeromod/4(yad1)
  massinit/1 -> Aero axes-cg transformation/5(massinit), Gust axes-cg transformation/3(massinit), Aeromod/3(massinit)
  Aeromod/1(Ca) -> Aero axes-cg transformation/1(Ca model)
  Aeromod/2(Cadot) -> Aero axes-cg transformation/2(Cadot model)
  Aeromod/3(Cbdot) -> Aero axes-cg transformation/3(Cbdot model)
  Aeromod/4(Cag) -> Gust axes-cg transformation/1(Cag model)
  x/1 -> Aero axes-cg transformation/4("x "), Gust axes-cg transformation/2("x "), FMaerodims/4(x), Aeromod/1(x)
  yatm/1 -> Aeromod/7(yatm)

== system Citation/Cessna Citation 500/Citation model DASMAT/AIRCRAFT MODEL/AIRDATA ==
  x : Inport
  terrain elevation : Inport  Port=2
  Demux : Demux  Outputs=[8 2 8]
  Demux1 : Demux  Outputs=[5 1 2]
  Mux : Mux  Inputs=[5 1 2]
  Sum : Sum  Inputs=-+|  SaturateOnIntegerOverflow=on
  airdata : S-Function  FunctionName=ac_atmos  SFunctionDeploymentMode=off  EnableBusSupport=off
  yatm : Outport
  yad1 : Outport  Port=2
  yad2 : Outport  Port=3
  wires:
  x/1 -> airdata/1
  airdata/1 -> Demux/1
  Demux/2 -> yad1/1
  Demux/3 -> yad2/1
  Demux/1 -> Demux1/1
  Mux/1 -> yatm/1
  Demux1/1 -> Mux/1
  Demux1/3 -> Mux/3
  Demux1/2 -> Sum/2
  Sum/1 -> Mux/2
  terrain elevation/1 -> Sum/1

== system Citation/Cessna Citation 500/Citation model DASMAT/AIRCRAFT MODEL/EFM ==
  x : Inport
  ut : Inport  Port=2
  massinit : Inport  Port=3
  yatm : Inport  Port=4
  yad1 : Inport  Port=5
  yad2 : Inport  Port=6
  Engine axes-cg transformation : Subsystem
  Engmod : Subsystem
  FMt : Outport
  ypp : Outport  Port=2
  wires:
  massinit/1 -> Engine axes-cg transformation/3(massinit)
  Engine axes-cg transformation/1(FMt) -> FMt/1
  ut/1 -> Engmod/2(ut)
  yatm/1 -> Engmod/3(yatm)
  yad2/1 -> Engmod/5(yad2)
  x/1 -> Engine axes-cg transformation/2("x "), Engmod/1(x)
  yad1/1 -> Engmod/4(yad1)
  Engmod/1(FMt) -> Engine axes-cg transformation/1(FMt model)
  Engmod/2(ypp) -> ypp/1

== system Citation/Cessna Citation 500/Citation model DASMAT/AIRCRAFT MODEL/EQM ==
  "FMtot " : Inport
  FMa : Inport  Port=2
  FMadot : Inport  Port=3
  FMbdot : Inport  Port=4
  massinit : Inport  Port=5
  wind : Inport  Port=6
  CFMa correction : Subsystem
  Integrator : Integrator  InitialCondition=x0
  State Derivatives : Subsystem
  x : Outport
  xdot : Outport  Port=2
  yuvw : Outport  Port=3
  FMtot corrected : Outport  Port=4
  FMa corrected : Outport  Port=5
  wires:
  State Derivatives/2(yuvw) -> yuvw/1
  State Derivatives/3(FMtot corrected) -> FMtot corrected/1
  FMa/1 -> CFMa correction/2(FMa)
  State Derivatives/1(xdot) -> xdot/1, CFMa correction/1(xdot), Integrator/1
  CFMa correction/1(FMa corrected) -> FMa corrected/1
  massinit/1 -> State Derivatives/5(massinit)
  "FMtot "/1 -> State Derivatives/2(FMtot)
  FMadot/1 -> CFMa correction/3(FMadot), State Derivatives/3(FMadot)
  FMbdot/1 -> CFMa correction/4(FMbdot), State Derivatives/4(FMbdot)
  Integrator/1 -> State Derivatives/1(x), x/1
  wind/1 -> State Derivatives/6(wind)

== system Citation/Cessna Citation 500/Citation model DASMAT/AIRCRAFT MODEL/FM SORT ==
  FMa : Inport
  FMag : Inport  Port=2
  FMt : Inport  Port=3
  "Fgr " : Inport  Port=4
  Fgear : Inport  Port=5
  Mux : Mux  Inputs=[12 12]
  Sum : Sum  Inputs=+++++  SaturateOnIntegerOverflow=on  InputSameDT=on  OutDataTypeStr=Inherit: Same as first input
  Sum1 : Sum  Inputs=++++  SaturateOnIntegerOverflow=on  InputSameDT=on  OutDataTypeStr=Inherit: Same as first input
  aero : Demux  Outputs=[12 12]
  engine : Demux  Outputs=[12 12]
  gear : Demux  Outputs=[12 12]
  gust : Demux  Outputs=[12 12]
  FMtot : Outport
  wires:
  FMt/1 -> engine/1
  FMa/1 -> aero/1
  FMag/1 -> gust/1
  gust/2 -> Sum1/2
  Sum1/1 -> Mux/2
  engine/2 -> Sum1/3
  aero/2 -> Sum1/1
  gust/1 -> Sum/2
  engine/1 -> Sum/3
  Sum/1 -> Mux/1
  "Fgr "/1 -> Sum/4
  aero/1 -> Sum/1
  Mux/1 -> FMtot/1
  Fgear/1 -> gear/1
  gear/1 -> Sum/5
  gear/2 -> Sum1/4

== system Citation/Cessna Citation 500/Citation model DASMAT/AIRCRAFT MODEL/GRAVITY ==
  "x " : Inport
  massinit : Inport  Port=2
  yatm : Inport  Port=3
  Fgr transformation : S-Function  FunctionName=ac_axes  Parameters=3  SFunctionDeploymentMode=off  EnableBusSupport=off
  Mux : Mux  Inputs=[12 3]
  Mux1 : Mux  Inputs=3
  Terminator_{1..9} (9 alike) : Terminator
  W : Product  SaturateOnIntegerOverflow=on  InputSameDT=on  OutDataTypeStr=Inherit: Same as first input
  atmosphere : Demux  Outputs=8
  mass cg inertia : Demux  Outputs=[1 3 4]
  zero : Constant  Value=0
  Fgr : Outport
  wires:
  mass cg inertia/3 -> Terminator_9/1
  mass cg inertia/2 -> Terminator_8/1
  atmosphere/8 -> Terminator_7/1
  atmosphere/7 -> Terminator_6/1
  atmosphere/6 -> Terminator_5/1
  atmosphere/5 -> Terminator_4/1
  atmosphere/3 -> Terminator_3/1
  atmosphere/2 -> Terminator_2/1
  atmosphere/1 -> Terminator_1/1
  Mux/1 -> Fgr transformation/1
  "x "/1 -> Mux/1
  Fgr transformation/1 -> Fgr/1
  mass cg inertia/1 -> W/1
  massinit/1 -> mass cg inertia/1
  yatm/1 -> atmosphere/1
  W/1 -> Mux1/3
  Mux1/1 -> Mux/2
  zero/1 -> Mux1/1, Mux1/2
  atmosphere/4 -> W/2

== system Citation/Cessna Citation 500/Citation model DASMAT/AIRCRAFT MODEL/LANDING GEAR ==
  note: Landing Gear Model
      | Cessna Citation 500
      | Version 0.04NLR
      | (c) A.R. Veldhuijzen September 2001
  x : Inport
  xdot : Inport  Port=2
  massinit : Inport  Port=3
  ua : Inport  Port=4
  terr elev : Inport  Port=5
  Gear axes-cg transformation : Subsystem
  Landing Gear model : Subsystem
  Switch : Switch  Threshold=0.95  SaturateOnIntegerOverflow=on
  gear position : Selector  IndexOptions=Index vector (dialog)  Indices=[8]  OutputSizes=1
  zero : Constant  Value=[0 0 0 0 0 0]
  Fmt : Outport
  wires:
  xdot/1 -> Landing Gear model/2(xdot)
  x/1 -> Landing Gear model/1(x), Gear axes-cg transformation/2("x ")
  massinit/1 -> Gear axes-cg transformation/3(massinit)
  Gear axes-cg transformation/1(FMt) -> Fmt/1
  zero/1 -> Switch/1
  Landing Gear model/1(Forces and Moments) -> Switch/3
  Switch/1 -> Gear axes-cg transformation/1(FMt model)
  ua/1 -> gear position/1
  gear position/1 -> Switch/2
  terr elev/1 -> Landing Gear model/3(terrain elevation)

== system Citation/Cessna Citation 500/Citation model DASMAT/AIRCRAFT MODEL/OBSERVATIONS ==
  note: Modified by Alex : Flight-Path Subsystem from Ac_mod instead of Ac_modpc
  x : Inport
  xdot : Inport  Port=2
  yuvw : Inport  Port=3
  FMtot : Inport  Port=4
  FMa : Inport  Port=5
  Fgr : Inport  Port=6
  massinit : Inport  Port=7
  yatm : Inport  Port=8
  Acceleration : Subsystem
  Energy : Subsystem
  Flight-Path : Subsystem
  yacc : Outport
  yfp : Outport  Port=2
  ys : Outport  Port=3
  wires:
  yuvw/1 -> Flight-Path/3(yuvw)
  Flight-Path/1(yfp) -> yfp/1
  Energy/1(ys) -> ys/1
  Acceleration/1(yacc) -> yacc/1
  FMa/1 -> Acceleration/4(FMa)
  Fgr/1 -> Acceleration/5(Fgr)
  yatm/1 -> Energy/3(yatm)
  FMtot/1 -> Acceleration/3(FMtot)
  Acceleration/2(acc earth) -> Flight-Path/4(acc earth)
  x/1 -> Flight-Path/1(x), Energy/1(x), Acceleration/1(x)
  xdot/1 -> Flight-Path/2(xdot), Energy/2(xdot), Acceleration/2(xdot)
  massinit/1 -> Acceleration/6(massinit)

== system Citation/Cessna Citation 500/Citation model DASMAT/AIRCRAFT MODEL/WIND//TURBULENCE ==
  "x " : Inport
  Logarithmic Wind model : Subsystem
  Mux : Mux  Inputs=[12 3]
  Vwind transformation : S-Function  FunctionName=ac_axes  Parameters=3  SFunctionDeploymentMode=off  EnableBusSupport=off
  wind : Outport
  wires:
  Mux/1 -> Vwind transformation/1
  Vwind transformation/1 -> wind/1
  "x "/1 -> Mux/1, Logarithmic Wind model/1(In1)
  Logarithmic Wind model/1(Out1) -> Mux/2

== system Citation/Cessna Citation 500/Controllers/NDI rotational rate controller/Linear Controller ==
  e_omega : Inport
  Demux : Demux  Outputs=3
  Integrator : Integrator
  Integrator1 : Integrator
  Integrator2 : Integrator
  Mux : Mux  Inputs=3
  PID Controller : simulink/Continuous/PID Controller  Controller=PID  TimeDomain=Continuous-time  SampleTime=-1  IntegratorMethod=Forward Euler  FilterMethod=Forward Euler  Form=Parallel  UseFilter=on  ControllerParametersSource=internal  P=10  I=1  D=0  N=100  InitialConditionSource=internal  InitialConditionForIntegrator=0  InitialConditionForFilter=0  ExternalReset=none  LimitOutput=off  UpperSaturationLimit=inf  LowerSaturationLimit=-inf  LinearizeAsGain=on  AntiWindupMode=none  Kb=1  TrackingMode=off  Kt=1  PParamMin=[]  PParamMax=[]  IParamMin=[]  IParamMax=[]  DParamMin=[]  DParamMax=[]  NParamMin=[]  NParamMax=[]  KbParamMin=[]  KbParamMax=[]  KtParamMin=[]  KtParamMax=[]  POutMin=[]  POutMax=[]  IOutMin=[]  IOutMax=[]  DOutMin=[]  DOutMax=[]  NOutMin=[]  NOutMax=[]  KbOutMin=[]  KbOutMax=[]  KtOutMin=[]  KtOutMax=[]  IntegratorOutMin=[]  IntegratorOutMax=[]  FilterOutMin=[]  FilterOutMax=[]  SumOutMin=[]  SumOutMax=[]  SumI1OutMin=[]  SumI1OutMax=[]  SumI2OutMin=[]  SumI2OutMax=[]  SumI3OutMin=[]  SumI3OutMax=[]  SumDOutMin=[]  SumDOutMax=[]  SaturationOutMin=[]  SaturationOutMax=[]  IntegratorContinuousStateAttributes=''  IntegratorStateMustResolveToSignalObject=off  IntegratorRTWStateStorageClass=Auto  FilterContinuousStateAttributes=''  FilterStateMustResolveToSignalObject=off  FilterRTWStateStorageClass=Auto  DifferentiatorICPrevScaledInput=0  DifferentiatorOutMin=[]  DifferentiatorOutMax=[]  FilterDiffOutCoefMin=[]  FilterDiffOutCoefMax=[]  SumDenOutMin=[]  SumDenOutMax=[]  SumNumOutMin=[]  SumNumOutMax=[]  ReciprocalOutMin=[]  ReciprocalOutMax=[]  DivideOutMin=[]  DivideOutMax=[]  TunerSelectOption=Transfer Function Based (PID Tuner App)
  PID Controller1 : simulink/Continuous/PID Controller  Controller=PID  TimeDomain=Continuous-time  SampleTime=-1  IntegratorMethod=Forward Euler  FilterMethod=Forward Euler  Form=Parallel  UseFilter=on  ControllerParametersSource=internal  P=5  I=1  D=0  N=100  InitialConditionSource=internal  InitialConditionForIntegrator=0  InitialConditionForFilter=0  ExternalReset=none  LimitOutput=off  UpperSaturationLimit=inf  LowerSaturationLimit=-inf  LinearizeAsGain=on  AntiWindupMode=none  Kb=1  TrackingMode=off  Kt=1  PParamMin=[]  PParamMax=[]  IParamMin=[]  IParamMax=[]  DParamMin=[]  DParamMax=[]  NParamMin=[]  NParamMax=[]  KbParamMin=[]  KbParamMax=[]  KtParamMin=[]  KtParamMax=[]  POutMin=[]  POutMax=[]  IOutMin=[]  IOutMax=[]  DOutMin=[]  DOutMax=[]  NOutMin=[]  NOutMax=[]  KbOutMin=[]  KbOutMax=[]  KtOutMin=[]  KtOutMax=[]  IntegratorOutMin=[]  IntegratorOutMax=[]  FilterOutMin=[]  FilterOutMax=[]  SumOutMin=[]  SumOutMax=[]  SumI1OutMin=[]  SumI1OutMax=[]  SumI2OutMin=[]  SumI2OutMax=[]  SumI3OutMin=[]  SumI3OutMax=[]  SumDOutMin=[]  SumDOutMax=[]  SaturationOutMin=[]  SaturationOutMax=[]  IntegratorContinuousStateAttributes=''  IntegratorStateMustResolveToSignalObject=off  IntegratorRTWStateStorageClass=Auto  FilterContinuousStateAttributes=''  FilterStateMustResolveToSignalObject=off  FilterRTWStateStorageClass=Auto  DifferentiatorICPrevScaledInput=0  DifferentiatorOutMin=[]  DifferentiatorOutMax=[]  FilterDiffOutCoefMin=[]  FilterDiffOutCoefMax=[]  SumDenOutMin=[]  SumDenOutMax=[]  SumNumOutMin=[]  SumNumOutMax=[]  ReciprocalOutMin=[]  ReciprocalOutMax=[]  DivideOutMin=[]  DivideOutMax=[]  TunerSelectOption=Transfer Function Based (PID Tuner App)
  PID Controller2 : simulink/Continuous/PID Controller  Controller=PID  TimeDomain=Continuous-time  SampleTime=-1  IntegratorMethod=Forward Euler  FilterMethod=Forward Euler  Form=Parallel  UseFilter=on  ControllerParametersSource=internal  P=10  I=1  D=0  N=100  InitialConditionSource=internal  InitialConditionForIntegrator=0  InitialConditionForFilter=0  ExternalReset=none  LimitOutput=off  UpperSaturationLimit=inf  LowerSaturationLimit=-inf  LinearizeAsGain=on  AntiWindupMode=none  Kb=1  TrackingMode=off  Kt=1  PParamMin=[]  PParamMax=[]  IParamMin=[]  IParamMax=[]  DParamMin=[]  DParamMax=[]  NParamMin=[]  NParamMax=[]  KbParamMin=[]  KbParamMax=[]  KtParamMin=[]  KtParamMax=[]  POutMin=[]  POutMax=[]  IOutMin=[]  IOutMax=[]  DOutMin=[]  DOutMax=[]  NOutMin=[]  NOutMax=[]  KbOutMin=[]  KbOutMax=[]  KtOutMin=[]  KtOutMax=[]  IntegratorOutMin=[]  IntegratorOutMax=[]  FilterOutMin=[]  FilterOutMax=[]  SumOutMin=[]  SumOutMax=[]  SumI1OutMin=[]  SumI1OutMax=[]  SumI2OutMin=[]  SumI2OutMax=[]  SumI3OutMin=[]  SumI3OutMax=[]  SumDOutMin=[]  SumDOutMax=[]  SaturationOutMin=[]  SaturationOutMax=[]  IntegratorContinuousStateAttributes=''  IntegratorStateMustResolveToSignalObject=off  IntegratorRTWStateStorageClass=Auto  FilterContinuousStateAttributes=''  FilterStateMustResolveToSignalObject=off  FilterRTWStateStorageClass=Auto  DifferentiatorICPrevScaledInput=0  DifferentiatorOutMin=[]  DifferentiatorOutMax=[]  FilterDiffOutCoefMin=[]  FilterDiffOutCoefMax=[]  SumDenOutMin=[]  SumDenOutMax=[]  SumNumOutMin=[]  SumNumOutMax=[]  ReciprocalOutMin=[]  ReciprocalOutMax=[]  DivideOutMin=[]  DivideOutMax=[]  TunerSelectOption=Transfer Function Based (PID Tuner App)
  Sum : Sum  Inputs=|+-
  Sum1 : Sum  Inputs=|+-
  Sum2 : Sum  Inputs=|+-
  v : Outport
  wires:
  Integrator1/1 -> Sum1/2  "p"
  Sum1/1 -> PID Controller1/1
  Integrator2/1 -> Sum2/2  "r"
  Integrator/1 -> Sum/2  "q"
  PID Controller2/1 -> Mux/3, Integrator2/1  "vr"
  PID Controller/1 -> Mux/2, Integrator/1  "vq"
  Sum2/1 -> PID Controller2/1
  PID Controller1/1 -> Mux/1, Integrator1/1  "vp"
  Sum/1 -> PID Controller/1
  Mux/1 -> v/1
  e_omega/1 -> Demux/1
  Demux/1 -> Sum1/1
  Demux/2 -> Sum/1
  Demux/3 -> Sum2/1

== system Citation/Pilot/Joystick/DualShock/Add deadzone  ==
  note: Add or subtract deadzone value
  note: Check sign
  "Value " : Inport
  "Input " : Inport  Port=2
  Product : Product
  Sign : Signum
  Sum4 : Sum  Inputs=|++
  Out1 : Outport
  wires:
  "Input "/1 -> Sign/1, Sum4/2
  Product/1 -> Sum4/1
  "Value "/1 -> Product/1
  Sum4/1 -> Out1/1
  Sign/1 -> Product/2

== system Citation/Pilot/Joystick/DualShock/Add deadzone 1 ==
  note: Check sign
  note: Add or subtract deadzone value
  "Value " : Inport
  "Input " : Inport  Port=2
  Product : Product
  Sign : Signum
  Sum4 : Sum  Inputs=|++
  Out1 : Outport
  wires:
  Sign/1 -> Product/2
  Sum4/1 -> Out1/1
  "Value "/1 -> Product/1
  Product/1 -> Sum4/1
  "Input "/1 -> Sum4/2, Sign/1

== system Citation/Pilot/Joystick/DualShock/Add deadzone 2 ==
  note: Add or subtract deadzone value
  note: Check sign
  "Value " : Inport
  "Input " : Inport  Port=2
  Product : Product
  Sign : Signum
  Sum4 : Sum  Inputs=|++
  Out1 : Outport
  wires:
  "Input "/1 -> Sign/1, Sum4/2
  Product/1 -> Sum4/1
  "Value "/1 -> Product/1
  Sum4/1 -> Out1/1
  Sign/1 -> Product/2

== system Citation/Pilot/Joystick/DualShock/Add deadzone 3 ==
  note: Check sign
  note: Add or subtract deadzone value
  "Value " : Inport
  "Input " : Inport  Port=2
  Product : Product
  Sign : Signum
  Sum4 : Sum  Inputs=|++
  Out1 : Outport
  wires:
  Sign/1 -> Product/2
  Sum4/1 -> Out1/1
  "Value "/1 -> Product/1
  Product/1 -> Sum4/1
  "Input "/1 -> Sum4/2, Sign/1

== system Citation/Pilot/Joystick/Logitech 3D Pro/Add deadzone  ==
  note: Add or subtract deadzone value
  note: Check sign
  "Value " : Inport
  "Input " : Inport  Port=2
  Product : Product
  Sign : Signum
  Sum4 : Sum  Inputs=|++
  Out1 : Outport
  wires:
  "Input "/1 -> Sign/1, Sum4/2
  Product/1 -> Sum4/1
  "Value "/1 -> Product/1
  Sum4/1 -> Out1/1
  Sign/1 -> Product/2

== system Citation/Pilot/Joystick/Logitech 3D Pro/Add deadzone 1 ==
  note: Check sign
  note: Add or subtract deadzone value
  "Value " : Inport
  "Input " : Inport  Port=2
  Product : Product
  Sign : Signum
  Sum4 : Sum  Inputs=|++
  Out1 : Outport
  wires:
  Sign/1 -> Product/2
  Sum4/1 -> Out1/1
  "Value "/1 -> Product/1
  Product/1 -> Sum4/1
  "Input "/1 -> Sum4/2, Sign/1

== system Citation/Pilot/Joystick/Logitech 3D Pro/Add deadzone 2 ==
  note: Add or subtract deadzone value
  note: Check sign
  "Value " : Inport
  "Input " : Inport  Port=2
  Product : Product
  Sign : Signum
  Sum4 : Sum  Inputs=|++
  Out1 : Outport
  wires:
  "Input "/1 -> Sign/1, Sum4/2
  Product/1 -> Sum4/1
  "Value "/1 -> Product/1
  Sum4/1 -> Out1/1
  Sign/1 -> Product/2

== system Citation/Pilot/Joystick/Logitech 3D Pro/Add deadzone 3 ==
  note: Check sign
  note: Add or subtract deadzone value
  "Value " : Inport
  "Input " : Inport  Port=2
  Product : Product
  Sign : Signum
  Sum4 : Sum  Inputs=|++
  Out1 : Outport
  wires:
  Sign/1 -> Product/2
  Sum4/1 -> Out1/1
  "Value "/1 -> Product/1
  Product/1 -> Sum4/1
  "Input "/1 -> Sum4/2, Sign/1
